simulink library "inductance"  (R2024a)
settings: Solver=VariableStepAuto  StartTime=0.0  StopTime=10.0  RelTol=1e-3
undefined symbols (not defined in the file): a
settings Model: Creator=Bocchio  LastModifiedBy=Bocchio

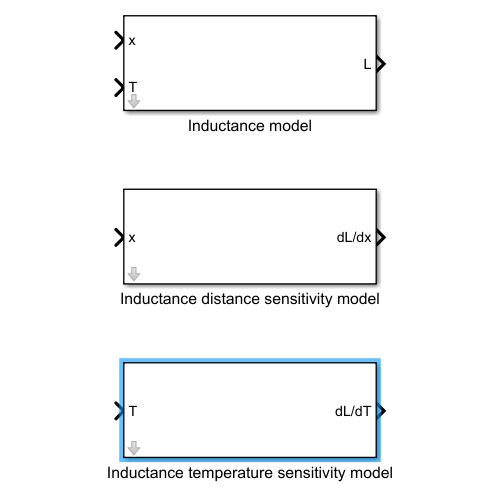
[thumbnail: Simulink's stored preview of the top-level diagram]
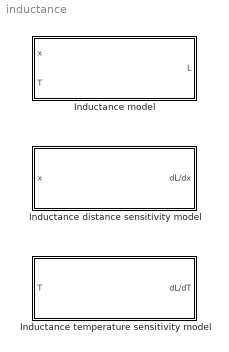
== system inductance ==
  Inductance distance sensitivity model : Subsystem  mask{Lx=0, a=a}
      mask DialogControl DescGroupVar Prompt: Inductance sensitivity to object distance
      mask DialogControl DescTextVar Prompt: Insert the parameters of the inductor
  Inductance model : Subsystem  mask(Inductance model){L0=0, Lx=0, a=a}
      mask DialogControl DescGroupVar Prompt: Inductance model
      mask DialogControl DescTextVar Prompt: Insert the parameters of the inductance
  Inductance temperature sensitivity model : Subsystem
      mask DialogControl DescGroupVar Prompt: Inductance sensitivity to object temperature
      mask DialogControl DescTextVar Prompt: Still to be determined. For now dL/dT = 0

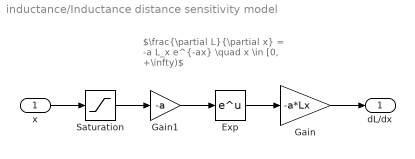
== system inductance/Inductance distance sensitivity model ==
  note: $\frac{\partial L}{\partial x} = -a L_x e^{-ax} \quad x \in [0, +\infty)$
  x : Inport
  Exp : Math
  Gain : Gain  Gain=-a*Lx
  Gain1 : Gain  Gain=-a
  Saturation : Saturate  UpperLimit=+inf  LowerLimit=0
  dL/dx : Outport
  wires:
  Gain1/1 -> Exp/1
  Exp/1 -> Gain/1
  x/1 -> Saturation/1
  Gain/1 -> dL/dx/1
  Saturation/1 -> Gain1/1

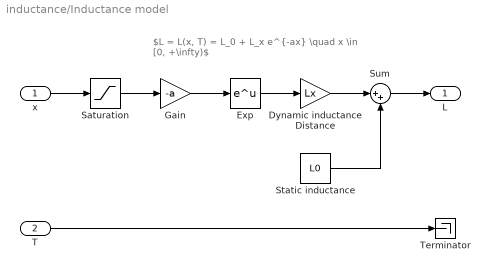
== system inductance/Inductance model ==
  note: $L = L(x, T) = L_0 + L_x e^{-ax} \quad x \in [0, +\infty)$
  x : Inport
  T : Inport  Port=2
  Dynamic inductance Distance : Gain  Gain=Lx
  Exp : Math
  Gain : Gain  Gain=-a
  Saturation : Saturate  UpperLimit=+inf  LowerLimit=0
  Static inductance : Constant  Value=L0
  Sum : Sum  Inputs=|++
  Terminator : Terminator
  L : Outport
  wires:
  Sum/1 -> L/1
  Dynamic inductance Distance/1 -> Sum/1
  Static inductance/1 -> Sum/2
  Exp/1 -> Dynamic inductance Distance/1
  Gain/1 -> Exp/1
  x/1 -> Saturation/1
  T/1 -> Terminator/1
  Saturation/1 -> Gain/1

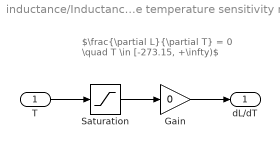
== system inductance/Inductance temperature sensitivity model ==
  note: $\frac{\partial L}{\partial T} = 0 \quad T \in [-273.15, +\infty)$
  T : Inport
  Gain : Gain  Gain=0
  Saturation : Saturate  UpperLimit=+inf  LowerLimit=-273.15
  dL/dT : Outport
  wires:
  Gain/1 -> dL/dT/1
  T/1 -> Saturation/1
  Saturation/1 -> Gain/1
